simulink model "w3_warplab_trigger_proc"  (Simulink 7.7)
settings: Solver=ode45  StartTime=0.0  StopTime=100  RelTol=1e-3
InitFcn:
  | warplab_trigger_proc_init
StartFcn:
  | warplab_trigger_proc_init
undefined symbols (not defined in the file or in its folder): gcbh, xlBlockLoadCallback, xlGetNormalizedPeriod
libraries: xbsIndex_r4 x817, xbsEDKLib_r4 x1
(part 5 of 6)

== system w3_warplab_trigger_proc/Trigger Sources/Energy ==
  16LSB : xbsIndex_r4/Slice  nbits=16  boolean_output=off  mode=Lower Bit Location + Width  bit1=0  base1=MSB of Input  bit0=0  base0=LSB of Input  dbl_ovrd=off  block_type=slice
  16MSB : xbsIndex_r4/Slice  nbits=16  boolean_output=off  mode=Lower Bit Location + Width  bit1=0  base1=MSB of Input  bit0=16  base0=LSB of Input  dbl_ovrd=off  block_type=slice
  AntA Detector : Subsystem
  AntB Detector : Subsystem
  AntC Detector : Subsystem
  AntD Detector : Subsystem
  Convert : xbsIndex_r4/Convert  gui_display_data_type=Boolean  arith_type=Boolean  n_bits=16  bin_pt=14  float_type=Single  exp_bits=8  fraction_bits=24  quantization=Truncate  overflow=Wrap  en=off  latency=0  dbl_ovrd=off  pipeline=off  block_type=convert
  MIMO Logic : Subsystem
  Posedge : Subsystem
  RFA_RSSI : xbsIndex_r4/Gateway In  gui_display_data_type=Fixed-point  arith_type=Unsigned  n_bits=10  bin_pt=0  preci_type=Single  exp_width=8  frac_width=24  quantization=Truncate  overflow=Wrap  period=1  dbl_ovrd=off  timing_constraint=None  locs_specified=off  LOCs={}  UseAsADC=off  ADCChannel='1'  inherit_from_input=off  hdl_port=on  block_type=gatewayin
      settings: block_version=VER_STRING_GOES_HERE
  RFB_RSSI : xbsIndex_r4/Gateway In  gui_display_data_type=Fixed-point  arith_type=Unsigned  n_bits=10  bin_pt=0  preci_type=Single  exp_width=8  frac_width=24  quantization=Truncate  overflow=Wrap  period=1  dbl_ovrd=off  timing_constraint=None  locs_specified=off  LOCs={}  UseAsADC=off  ADCChannel='1'  inherit_from_input=off  hdl_port=on  block_type=gatewayin
      settings: infoedit="Gateway in block.  Converts inputs of type Simulink integer, double and fixed point to  Xilinx fixed point type.<P><P>Hardware notes:  In hardware these blocks become top level input ports."  block_version=VER_STRING_GOES_HERE
  RFC_RSSI : xbsIndex_r4/Gateway In  gui_display_data_type=Fixed-point  arith_type=Unsigned  n_bits=10  bin_pt=0  preci_type=Single  exp_width=8  frac_width=24  quantization=Truncate  overflow=Wrap  period=1  dbl_ovrd=off  timing_constraint=None  locs_specified=off  LOCs={}  UseAsADC=off  ADCChannel='1'  inherit_from_input=off  hdl_port=on  block_type=gatewayin
      settings: infoedit="Gateway in block.  Converts inputs of type Simulink integer, double and fixed point to  Xilinx fixed point type.<P><P>Hardware notes:  In hardware these blocks become top level input ports."  block_version=VER_STRING_GOES_HERE
  RFD_RSSI : xbsIndex_r4/Gateway In  gui_display_data_type=Fixed-point  arith_type=Unsigned  n_bits=10  bin_pt=0  preci_type=Single  exp_width=8  frac_width=24  quantization=Truncate  overflow=Wrap  period=1  dbl_ovrd=off  timing_constraint=None  locs_specified=off  LOCs={}  UseAsADC=off  ADCChannel='1'  inherit_from_input=off  hdl_port=on  block_type=gatewayin
      settings: infoedit="Gateway in block.  Converts inputs of type Simulink integer, double and fixed point to  Xilinx fixed point type.<P><P>Hardware notes:  In hardware these blocks become top level input ports."  block_version=VER_STRING_GOES_HERE
  RSSI_CLK : xbsIndex_r4/Gateway In  gui_display_data_type=Boolean  arith_type=Boolean  n_bits=10  bin_pt=0  preci_type=Single  exp_width=8  frac_width=24  quantization=Truncate  overflow=Wrap  period=1  dbl_ovrd=off  timing_constraint=None  locs_specified=off  LOCs={}  UseAsADC=off  ADCChannel='1'  inherit_from_input=off  hdl_port=on  block_type=gatewayin
      settings: block_version=VER_STRING_GOES_HERE
  b0 : xbsIndex_r4/Slice  nbits=1  boolean_output=off  mode=Lower Bit Location + Width  bit1=0  base1=MSB of Input  bit0=0  base0=LSB of Input  dbl_ovrd=off  block_type=slice
  b1 : xbsIndex_r4/Slice  nbits=1  boolean_output=off  mode=Lower Bit Location + Width  bit1=0  base1=MSB of Input  bit0=1  base0=LSB of Input  dbl_ovrd=off  block_type=slice
  b2 : xbsIndex_r4/Slice  nbits=1  boolean_output=off  mode=Lower Bit Location + Width  bit1=0  base1=MSB of Input  bit0=2  base0=LSB of Input  dbl_ovrd=off  block_type=slice
  b3 : xbsIndex_r4/Slice  nbits=1  boolean_output=off  mode=Lower Bit Location + Width  bit1=0  base1=MSB of Input  bit0=3  base0=LSB of Input  dbl_ovrd=off  block_type=slice
  b4 : xbsIndex_r4/Slice  nbits=1  boolean_output=off  mode=Lower Bit Location + Width  bit1=0  base1=MSB of Input  bit0=4  base0=LSB of Input  dbl_ovrd=off  block_type=slice
  b5 : xbsIndex_r4/Slice  nbits=1  boolean_output=off  mode=Lower Bit Location + Width  bit1=0  base1=MSB of Input  bit0=5  base0=LSB of Input  dbl_ovrd=off  block_type=slice
  b[15:8] : xbsIndex_r4/Slice  nbits=8  boolean_output=off  mode=Lower Bit Location + Width  bit1=0  base1=MSB of Input  bit0=8  base0=LSB of Input  dbl_ovrd=off  block_type=slice
  b[20:16] : xbsIndex_r4/Slice  nbits=5  boolean_output=off  mode=Lower Bit Location + Width  bit1=0  base1=MSB of Input  bit0=16  base0=LSB of Input  dbl_ovrd=off  block_type=slice
  b[7:0] : xbsIndex_r4/Slice  nbits=8  boolean_output=off  mode=Lower Bit Location + Width  bit1=0  base1=MSB of Input  bit0=0  base0=LSB of Input  dbl_ovrd=off  block_type=slice
  Trigger : Outport
  tag scope: pktDetMask_A=global, pktDetMask_B=global, pktDetMask_C=global, pktDetMask_D=global, pktDetReset=global, pktDet_duration_busy=global, pktDet_duration_idle=global, pktDet_energyThresh_busy=global, pktDet_energyThresh_idle=global, regPktDet_RSSIavgLength=global
  wires:
  AntA Detector/1(pktdet) -> MIMO Logic/1(Det A)
  [pktDetReset] -> Convert/1
  RFA_RSSI/1 -> AntA Detector/1(RSSI)
  [reg_pkt_det_config] -> b0/1, b1/1, b2/1, b3/1, b4/1, b5/1
  b0/1 -> [pktDetReset]
  b2/1 -> [pktDetMask_A]
  b3/1 -> [pktDetMask_B]
  [reg_pkt_det_thresh] -> 16LSB/1, 16MSB/1
  [reg_pkt_det_duration] -> b[7:0]/1, b[15:8]/1, b[20:16]/1
  16LSB/1 -> [pktDet_energyThresh_idle]
  16MSB/1 -> [pktDet_energyThresh_busy]
  b[7:0]/1 -> [pktDet_duration_idle]
  b[15:8]/1 -> [pktDet_duration_busy]
  b[20:16]/1 -> [regPktDet_RSSIavgLength]
  AntB Detector/1(pktdet) -> MIMO Logic/2(Det B)
  AntC Detector/1(pktdet) -> MIMO Logic/3(Det C)
  AntD Detector/1(pktdet) -> MIMO Logic/4(Det D)
  RFB_RSSI/1 -> AntB Detector/1(RSSI)
  RFC_RSSI/1 -> AntC Detector/1(RSSI)
  RFD_RSSI/1 -> AntD Detector/1(RSSI)
  Convert/1 -> AntA Detector/2(Reset), AntB Detector/2(Reset), AntC Detector/2(Reset), AntD Detector/2(Reset)
  b4/1 -> [pktDetMask_C]
  b5/1 -> [pktDetMask_D]
  MIMO Logic/1(PktDet) -> Trigger/1
  RSSI_CLK/1 -> Posedge/1(D)
  Posedge/1(Q) -> AntC Detector/3(En), AntD Detector/3(En), AntB Detector/3(En), AntA Detector/3(En)

== system w3_warplab_trigger_proc/Trigger Sources/Ethernet ==
  AXI_STR_TDATA : xbsIndex_r4/Gateway In  gui_display_data_type=Fixed-point  arith_type=Unsigned  n_bits=32  bin_pt=0  preci_type=Single  exp_width=8  frac_width=24  quantization="Round  (unbiased: +/- Inf)"  overflow=Wrap  period=1  dbl_ovrd=off  timing_constraint=None  locs_specified=off  LOCs={}  UseAsADC=off  ADCChannel='1'  inherit_from_input=off  hdl_port=on  block_type=gatewayin
  AXI_STR_TDEST : xbsIndex_r4/Gateway In  gui_display_data_type=Fixed-point  arith_type=Unsigned  n_bits=4  bin_pt=0  preci_type=Single  exp_width=8  frac_width=24  quantization="Round  (unbiased: +/- Inf)"  overflow=Wrap  period=1  dbl_ovrd=off  timing_constraint=None  locs_specified=off  LOCs={}  UseAsADC=off  ADCChannel='1'  inherit_from_input=off  hdl_port=on  block_type=gatewayin
  AXI_STR_TKEEP : xbsIndex_r4/Gateway In  gui_display_data_type=Fixed-point  arith_type=Unsigned  n_bits=4  bin_pt=0  preci_type=Single  exp_width=8  frac_width=24  quantization="Round  (unbiased: +/- Inf)"  overflow=Wrap  period=1  dbl_ovrd=off  timing_constraint=None  locs_specified=off  LOCs={}  UseAsADC=off  ADCChannel='1'  inherit_from_input=off  hdl_port=on  block_type=gatewayin
  AXI_STR_TLAST : xbsIndex_r4/Gateway In  gui_display_data_type=Fixed-point  arith_type=Unsigned  n_bits=1  bin_pt=0  preci_type=Single  exp_width=8  frac_width=24  quantization="Round  (unbiased: +/- Inf)"  overflow=Wrap  period=1  dbl_ovrd=off  timing_constraint=None  locs_specified=off  LOCs={}  UseAsADC=off  ADCChannel='1'  inherit_from_input=off  hdl_port=on  block_type=gatewayin
  AXI_STR_TREADY : xbsIndex_r4/Gateway In  gui_display_data_type=Fixed-point  arith_type=Unsigned  n_bits=1  bin_pt=0  preci_type=Single  exp_width=8  frac_width=24  quantization="Round  (unbiased: +/- Inf)"  overflow=Wrap  period=1  dbl_ovrd=off  timing_constraint=None  locs_specified=off  LOCs={}  UseAsADC=off  ADCChannel='1'  inherit_from_input=off  hdl_port=on  block_type=gatewayin
  AXI_STR_TSTRB : xbsIndex_r4/Gateway In  gui_display_data_type=Fixed-point  arith_type=Unsigned  n_bits=4  bin_pt=0  preci_type=Single  exp_width=8  frac_width=24  quantization="Round  (unbiased: +/- Inf)"  overflow=Wrap  period=1  dbl_ovrd=off  timing_constraint=None  locs_specified=off  LOCs={}  UseAsADC=off  ADCChannel='1'  inherit_from_input=off  hdl_port=on  block_type=gatewayin
  AXI_STR_TVALID : xbsIndex_r4/Gateway In  gui_display_data_type=Fixed-point  arith_type=Unsigned  n_bits=1  bin_pt=0  preci_type=Single  exp_width=8  frac_width=24  quantization="Round  (unbiased: +/- Inf)"  overflow=Wrap  period=1  dbl_ovrd=off  timing_constraint=None  locs_specified=off  LOCs={}  UseAsADC=off  ADCChannel='1'  inherit_from_input=off  hdl_port=on  block_type=gatewayin
  Constant{,1..4,6..7} (7 alike) : Constant  Value=0
  Pkt Comp : Subsystem
  Terminator : Terminator
  Terminator1 : Terminator
  Terminator2 : Terminator
  Trigger : Outport
  wires:
  Constant/1 -> AXI_STR_TVALID/1
  Constant1/1 -> AXI_STR_TDATA/1
  Constant2/1 -> AXI_STR_TLAST/1
  Constant3/1 -> AXI_STR_TSTRB/1
  AXI_STR_TVALID/1 -> Pkt Comp/1(TVALID)  "TVALID"
  AXI_STR_TDATA/1 -> Pkt Comp/2(TDATA)  "TDATA"
  AXI_STR_TREADY/1 -> Pkt Comp/3(TREADY)  "TREADY"
  Constant4/1 -> AXI_STR_TREADY/1
  AXI_STR_TLAST/1 -> Pkt Comp/4(TLAST)  "TLAST"
  Constant6/1 -> AXI_STR_TKEEP/1
  Constant7/1 -> AXI_STR_TDEST/1
  AXI_STR_TDEST/1 -> Terminator2/1  "TDEST"
  AXI_STR_TKEEP/1 -> Terminator1/1  "TKEEP"
  AXI_STR_TSTRB/1 -> Terminator/1  "TSTRB"
  Pkt Comp/1(Trigger) -> Trigger/1

== system w3_warplab_trigger_proc/Trigger Sources/Software ==
  Trigger : Outport
  wires:
  [Software_Trig] -> Trigger/1

== system w3_warplab_trigger_proc/Trigger Sources/Energy/AntA Detector ==
  RSSI : Inport
  Reset : Inport  Port=2
  En : Inport  Port=3
  ASR : xbsIndex_r4/Addressable Shift Register  infer_latency=on  depth=2  initVector=[0]  en=on  dbl_ovrd=off  use_behavioral_HDL=off  Optimization=Resource  use_rpm=off  block_type=addrsr
      settings: infoedit="Delay of configurable length.  Any element in the delay line can be addressed and driven onto the output port.<br><br>Hardware notes: This block is implemented using SRL16s. If Virtex-4 or Spartan-3 device is used, multiple SRLC16s are cascaded together."  block_version=VER_STRING_GOES_HERE
  Busy Detection : Subsystem
  Delay : xbsIndex_r4/Delay  rst=off  infoeditControl=Selection of Reset will increase slice count due to use of real FFs and instead of SRLs  en=off  latency=2  dbl_ovrd=off  reg_retiming=off  block_type=delay
  Gateway Out{,1..5} (6 alike) : xbsIndex_r4/Gateway Out  inherit_from_input=off  hdl_port=off  timing_constraint=None  locs_specified=off  LOCs={}  UseAsDAC=off  DACChannel='1'  block_type=gatewayout
      settings: infoedit="Gateway out block.  Converts Xilinx fixed point inputs into ouputs of type Simulink integer, double, or fixed point.<P><P>Hardware notes:  In hardware these blocks become top level output ports or are discarded, depending on how they are configured."  block_version=8.2
  Idle Detection : Subsystem
  Logical : xbsIndex_r4/Logical  logical_function=AND  inputs=2  en=off  latency=0  precision=Full  arith_type=Unsigned  n_bits=16  bin_pt=0  align_bp=on  dbl_ovrd=off  block_type=logical
  Pkt Det Decision : Scope  NumInputPorts=6
      settings: TimeRange=1000  YMin=0~0~0~0~0~0  YMax=1000~15000~1~1~1~1
  Running Sum : Subsystem
  pktdet : Outport
  wires:
  Reset/1 -> Running Sum/2(reset), Idle Detection/2(Reset), Busy Detection/2(Reset)
  [regPktDet_RSSIavgLength] -> Running Sum/3(avglen)
  Gateway Out/1 -> Pkt Det Decision/1  "RAWRSSI"
  Gateway Out1/1 -> Pkt Det Decision/2  "AVGRSSI"
  Gateway Out2/1 -> Pkt Det Decision/3  "IDLE"
  RSSI/1 -> Running Sum/1(RSSI), Gateway Out/1
  Running Sum/1(avg) -> Idle Detection/1(Avg RSSI), Busy Detection/1(Avg RSSI), Gateway Out1/1
  Idle Detection/1(Idle) -> Gateway Out2/1, Delay/1
  [pktDet_duration_busy] -> ASR/2
  ASR/1 -> Logical/1, Gateway Out5/1
  Busy Detection/1(Busy) -> Logical/2, Gateway Out3/1
  Logical/1 -> pktdet/1, Gateway Out4/1
  Gateway Out3/1 -> Pkt Det Decision/5  "BUSY"
  Gateway Out4/1 -> Pkt Det Decision/6  "DET"
  Gateway Out5/1 -> Pkt Det Decision/4  "IDLE DLY"
  Delay/1 -> ASR/1
  En/1 -> Running Sum/4(en), ASR/3, Idle Detection/3(en), Busy Detection/3(en)

== system w3_warplab_trigger_proc/Trigger Sources/Energy/AntB Detector ==
  RSSI : Inport
  Reset : Inport  Port=2
  En : Inport  Port=3
  ASR : xbsIndex_r4/Addressable Shift Register  infer_latency=on  depth=2  initVector=[0]  en=on  dbl_ovrd=off  use_behavioral_HDL=off  Optimization=Resource  use_rpm=off  block_type=addrsr
      settings: infoedit="Delay of configurable length.  Any element in the delay line can be addressed and driven onto the output port.<br><br>Hardware notes: This block is implemented using SRL16s. If Virtex-4 or Spartan-3 device is used, multiple SRLC16s are cascaded together."  block_version=VER_STRING_GOES_HERE
  Busy Detection : Subsystem
  Delay : xbsIndex_r4/Delay  rst=off  infoeditControl=Selection of Reset will increase slice count due to use of real FFs and instead of SRLs  en=off  latency=2  dbl_ovrd=off  reg_retiming=off  block_type=delay
  Gateway Out{,1..5} (6 alike) : xbsIndex_r4/Gateway Out  inherit_from_input=off  hdl_port=off  timing_constraint=None  locs_specified=off  LOCs={}  UseAsDAC=off  DACChannel='1'  block_type=gatewayout
      settings: infoedit="Gateway out block.  Converts Xilinx fixed point inputs into ouputs of type Simulink integer, double, or fixed point.<P><P>Hardware notes:  In hardware these blocks become top level output ports or are discarded, depending on how they are configured."  block_version=8.2
  Idle Detection : Subsystem
  Logical : xbsIndex_r4/Logical  logical_function=AND  inputs=2  en=off  latency=0  precision=Full  arith_type=Unsigned  n_bits=16  bin_pt=0  align_bp=on  dbl_ovrd=off  block_type=logical
  Pkt Det Decision : Scope  NumInputPorts=6
      settings: TimeRange=1000  YMin=0~0~0~0~0~0  YMax=1000~15000~1~1~1~1
  Running Sum : Subsystem
  pktdet : Outport
  wires:
  En/1 -> ASR/3, Idle Detection/3(en), Busy Detection/3(en), Running Sum/4(en)
  Delay/1 -> ASR/1
  Gateway Out5/1 -> Pkt Det Decision/4  "IDLE DLY"
  Gateway Out4/1 -> Pkt Det Decision/6  "DET"
  Gateway Out3/1 -> Pkt Det Decision/5  "BUSY"
  Logical/1 -> Gateway Out4/1, pktdet/1
  Busy Detection/1(Busy) -> Gateway Out3/1, Logical/2
  ASR/1 -> Gateway Out5/1, Logical/1
  [pktDet_duration_busy] -> ASR/2
  Idle Detection/1(Idle) -> Delay/1, Gateway Out2/1
  Running Sum/1(avg) -> Gateway Out1/1, Idle Detection/1(Avg RSSI), Busy Detection/1(Avg RSSI)
  RSSI/1 -> Gateway Out/1, Running Sum/1(RSSI)
  Gateway Out2/1 -> Pkt Det Decision/3  "IDLE"
  Gateway Out1/1 -> Pkt Det Decision/2  "AVGRSSI"
  Gateway Out/1 -> Pkt Det Decision/1  "RAWRSSI"
  [regPktDet_RSSIavgLength] -> Running Sum/3(avglen)
  Reset/1 -> Idle Detection/2(Reset), Busy Detection/2(Reset), Running Sum/2(reset)

== system w3_warplab_trigger_proc/Trigger Sources/Energy/AntC Detector ==
  RSSI : Inport
  Reset : Inport  Port=2
  En : Inport  Port=3
  ASR : xbsIndex_r4/Addressable Shift Register  infer_latency=on  depth=2  initVector=[0]  en=on  dbl_ovrd=off  use_behavioral_HDL=off  Optimization=Resource  use_rpm=off  block_type=addrsr
      settings: infoedit="Delay of configurable length.  Any element in the delay line can be addressed and driven onto the output port.<br><br>Hardware notes: This block is implemented using SRL16s. If Virtex-4 or Spartan-3 device is used, multiple SRLC16s are cascaded together."  block_version=VER_STRING_GOES_HERE
  Busy Detection : Subsystem
  Delay : xbsIndex_r4/Delay  rst=off  infoeditControl=Selection of Reset will increase slice count due to use of real FFs and instead of SRLs  en=off  latency=2  dbl_ovrd=off  reg_retiming=off  block_type=delay
  Gateway Out{,1..5} (6 alike) : xbsIndex_r4/Gateway Out  inherit_from_input=off  hdl_port=off  timing_constraint=None  locs_specified=off  LOCs={}  UseAsDAC=off  DACChannel='1'  block_type=gatewayout
      settings: infoedit="Gateway out block.  Converts Xilinx fixed point inputs into ouputs of type Simulink integer, double, or fixed point.<P><P>Hardware notes:  In hardware these blocks become top level output ports or are discarded, depending on how they are configured."  block_version=8.2
  Idle Detection : Subsystem
  Logical : xbsIndex_r4/Logical  logical_function=AND  inputs=2  en=off  latency=0  precision=Full  arith_type=Unsigned  n_bits=16  bin_pt=0  align_bp=on  dbl_ovrd=off  block_type=logical
  Pkt Det Decision : Scope  NumInputPorts=6
      settings: TimeRange=1000  YMin=0~0~0~0~0~0  YMax=1000~15000~1~1~1~1
  Running Sum : Subsystem
  pktdet : Outport
  wires:
  Reset/1 -> Running Sum/2(reset), Busy Detection/2(Reset), Idle Detection/2(Reset)
  [regPktDet_RSSIavgLength] -> Running Sum/3(avglen)
  Gateway Out/1 -> Pkt Det Decision/1  "RAWRSSI"
  Gateway Out1/1 -> Pkt Det Decision/2  "AVGRSSI"
  Gateway Out2/1 -> Pkt Det Decision/3  "IDLE"
  RSSI/1 -> Running Sum/1(RSSI), Gateway Out/1
  Running Sum/1(avg) -> Busy Detection/1(Avg RSSI), Idle Detection/1(Avg RSSI), Gateway Out1/1
  Idle Detection/1(Idle) -> Gateway Out2/1, Delay/1
  [pktDet_duration_busy] -> ASR/2
  ASR/1 -> Logical/1, Gateway Out5/1
  Busy Detection/1(Busy) -> Logical/2, Gateway Out3/1
  Logical/1 -> pktdet/1, Gateway Out4/1
  Gateway Out3/1 -> Pkt Det Decision/5  "BUSY"
  Gateway Out4/1 -> Pkt Det Decision/6  "DET"
  Gateway Out5/1 -> Pkt Det Decision/4  "IDLE DLY"
  Delay/1 -> ASR/1
  En/1 -> Running Sum/4(en), ASR/3, Busy Detection/3(en), Idle Detection/3(en)

== system w3_warplab_trigger_proc/Trigger Sources/Energy/AntD Detector ==
  RSSI : Inport
  Reset : Inport  Port=2
  En : Inport  Port=3
  ASR : xbsIndex_r4/Addressable Shift Register  infer_latency=on  depth=2  initVector=[0]  en=on  dbl_ovrd=off  use_behavioral_HDL=off  Optimization=Resource  use_rpm=off  block_type=addrsr
      settings: infoedit="Delay of configurable length.  Any element in the delay line can be addressed and driven onto the output port.<br><br>Hardware notes: This block is implemented using SRL16s. If Virtex-4 or Spartan-3 device is used, multiple SRLC16s are cascaded together."  block_version=VER_STRING_GOES_HERE
  Busy Detection : Subsystem
  Delay : xbsIndex_r4/Delay  rst=off  infoeditControl=Selection of Reset will increase slice count due to use of real FFs and instead of SRLs  en=off  latency=2  dbl_ovrd=off  reg_retiming=off  block_type=delay
  Gateway Out{,1..5} (6 alike) : xbsIndex_r4/Gateway Out  inherit_from_input=off  hdl_port=off  timing_constraint=None  locs_specified=off  LOCs={}  UseAsDAC=off  DACChannel='1'  block_type=gatewayout
      settings: infoedit="Gateway out block.  Converts Xilinx fixed point inputs into ouputs of type Simulink integer, double, or fixed point.<P><P>Hardware notes:  In hardware these blocks become top level output ports or are discarded, depending on how they are configured."  block_version=8.2
  Idle Detection : Subsystem
  Logical : xbsIndex_r4/Logical  logical_function=AND  inputs=2  en=off  latency=0  precision=Full  arith_type=Unsigned  n_bits=16  bin_pt=0  align_bp=on  dbl_ovrd=off  block_type=logical
  Pkt Det Decision : Scope  NumInputPorts=6
      settings: TimeRange=1000  YMin=0~0~0~0~0~0  YMax=1000~15000~1~1~1~1
  Running Sum : Subsystem
  pktdet : Outport
  wires:
  En/1 -> ASR/3, Idle Detection/3(en), Busy Detection/3(en), Running Sum/4(en)
  Delay/1 -> ASR/1
  Gateway Out5/1 -> Pkt Det Decision/4  "IDLE DLY"
  Gateway Out4/1 -> Pkt Det Decision/6  "DET"
  Gateway Out3/1 -> Pkt Det Decision/5  "BUSY"
  Logical/1 -> Gateway Out4/1, pktdet/1
  Busy Detection/1(Busy) -> Gateway Out3/1, Logical/2
  ASR/1 -> Gateway Out5/1, Logical/1
  [pktDet_duration_busy] -> ASR/2
  Idle Detection/1(Idle) -> Delay/1, Gateway Out2/1
  Running Sum/1(avg) -> Gateway Out1/1, Idle Detection/1(Avg RSSI), Busy Detection/1(Avg RSSI)
  RSSI/1 -> Gateway Out/1, Running Sum/1(RSSI)
  Gateway Out2/1 -> Pkt Det Decision/3  "IDLE"
  Gateway Out1/1 -> Pkt Det Decision/2  "AVGRSSI"
  Gateway Out/1 -> Pkt Det Decision/1  "RAWRSSI"
  [regPktDet_RSSIavgLength] -> Running Sum/3(avglen)
  Reset/1 -> Idle Detection/2(Reset), Busy Detection/2(Reset), Running Sum/2(reset)

== system w3_warplab_trigger_proc/Trigger Sources/Energy/MIMO Logic ==
  Det A : Inport
  Det B : Inport  Port=2
  Det C : Inport  Port=3
  Det D : Inport  Port=4
  Convert{1..8} (8 alike) : xbsIndex_r4/Convert  gui_display_data_type=Fixed-point  arith_type=Unsigned  n_bits=1  bin_pt=0  float_type=Single  exp_bits=8  fraction_bits=24  quantization=Truncate  overflow=Flag as error  en=off  latency=0  dbl_ovrd=off  pipeline=off  block_type=convert
      settings: block_version=10.1.3
  Logical{,1,3..4} (4 alike) : xbsIndex_r4/Logical  logical_function=AND  inputs=2  en=off  latency=0  precision=Full  arith_type=Unsigned  n_bits=16  bin_pt=0  align_bp=on  dbl_ovrd=off  block_type=logical
  Logical2 : xbsIndex_r4/Logical  logical_function=OR  inputs=4  en=off  latency=0  precision=Full  arith_type=Unsigned  n_bits=16  bin_pt=0  align_bp=on  dbl_ovrd=off  block_type=logical
  PktDet : Outport
  wires:
  [pktDetMask_A] -> Convert2/1
  [pktDetMask_B] -> Convert3/1
  Det A/1 -> Convert7/1
  Det B/1 -> Convert1/1
  Convert7/1 -> Logical/1
  Convert2/1 -> Logical/2
  Convert1/1 -> Logical1/1
  Convert3/1 -> Logical1/2
  Logical/1 -> Logical2/1
  Logical1/1 -> Logical2/2
  Logical2/1 -> PktDet/1
  [pktDetMask_C] -> Convert5/1
  Det C/1 -> Convert4/1
  Convert4/1 -> Logical3/1
  Convert5/1 -> Logical3/2
  Logical3/1 -> Logical2/3
  [pktDetMask_D] -> Convert8/1
  Det D/1 -> Convert6/1
  Convert6/1 -> Logical4/1
  Convert8/1 -> Logical4/2
  Logical4/1 -> Logical2/4

== system w3_warplab_trigger_proc/Trigger Sources/Energy/Posedge ==
  D : Inport
  Delay : xbsIndex_r4/Delay  rst=off  infoeditControl=Selection of Reset will increase slice count due to use of real FFs and instead of SRLs  en=off  latency=1  dbl_ovrd=off  reg_retiming=off  block_type=delay
      settings: infoedit=Hardware notes: A delay line is a chain, each link of which is an SRL16 followed by a flip-flop. If register retiming is enabled, the delay line is a chain of flip-flops.  block_version=8.2
  Inverter : xbsIndex_r4/Inverter  en=off  latency=0  dbl_ovrd=off  block_type=inv
      settings: block_version=8.2
  Logical : xbsIndex_r4/Logical  logical_function=AND  inputs=2  en=off  latency=0  precision=Full  arith_type=Unsigned  n_bits=16  bin_pt=0  align_bp=on  dbl_ovrd=off  block_type=logical
      settings: block_version=8.2
  Q : Outport
  wires:
  D/1 -> Inverter/1, Logical/1
  Inverter/1 -> Delay/1
  Delay/1 -> Logical/2
  Logical/1 -> Q/1

== system w3_warplab_trigger_proc/Trigger Sources/Ethernet/Pkt Comp ==
  TVALID : Inport
  TDATA : Inport  Port=2
  TREADY : Inport  Port=3
  TLAST : Inport  Port=4
  Convert2 : xbsIndex_r4/Convert  gui_display_data_type=Boolean  arith_type=Boolean  n_bits=16  bin_pt=14  float_type=Single  exp_bits=8  fraction_bits=24  quantization=Truncate  overflow=Wrap  en=off  latency=0  dbl_ovrd=off  pipeline=off  block_type=convert
  Convert3 : xbsIndex_r4/Convert  gui_display_data_type=Boolean  arith_type=Boolean  n_bits=16  bin_pt=14  float_type=Single  exp_bits=8  fraction_bits=24  quantization=Truncate  overflow=Wrap  en=off  latency=0  dbl_ovrd=off  pipeline=off  block_type=convert
  Delay : xbsIndex_r4/Delay  rst=off  infoeditControl=Selection of Reset will increase slice count due to use of real FFs and instead of SRLs  en=off  latency=4  dbl_ovrd=off  reg_retiming=off  block_type=delay
  Delay1 : xbsIndex_r4/Delay  rst=off  infoeditControl=Selection of Reset will increase slice count due to use of real FFs and instead of SRLs  en=off  latency=3  dbl_ovrd=off  reg_retiming=off  block_type=delay
  Delay2 : xbsIndex_r4/Delay  rst=off  infoeditControl=Selection of Reset will increase slice count due to use of real FFs and instead of SRLs  en=off  latency=1  dbl_ovrd=off  reg_retiming=off  block_type=delay
  Delay3 : xbsIndex_r4/Delay  rst=off  infoeditControl=Selection of Reset will increase slice count due to use of real FFs and instead of SRLs  en=off  latency=1  dbl_ovrd=off  reg_retiming=off  block_type=delay
  Logical : xbsIndex_r4/Logical  logical_function=AND  inputs=2  en=off  latency=0  precision=Full  arith_type=Unsigned  n_bits=16  bin_pt=0  align_bp=on  dbl_ovrd=off  block_type=logical
  Output Reg 0 : Subsystem
  Pkt Match : Subsystem
  Pkt Word Addr : xbsIndex_r4/Counter  cnt_type=Count Limited  cnt_to=63  operation=Up  start_count=0  cnt_by_val=1  arith_type=Unsigned  n_bits=6  bin_pt=0  load_pin=off  rst=on  en=on  explicit_period=off  period=1  dbl_ovrd=off  use_behavioral_HDL=off  implementation=Fabric  block_type=counter
  Word Comp 0 : Subsystem
  Trigger : Outport
  tag scope: WordMatch_0=global
  wires:
  Logical/1 -> Convert2/1
  TVALID/1 -> Logical/1
  TREADY/1 -> Logical/2
  Pkt Word Addr/1 -> Word Comp 0/1(Word Addr)
  TLAST/1 -> Convert3/1
  Convert2/1 -> Pkt Word Addr/2, Delay3/1
  Convert3/1 -> Pkt Word Addr/1, Delay/1, Delay1/1
  TDATA/1 -> Delay2/1
  Delay/1 -> Pkt Match/3(Reset)
  Word Comp 0/1(Word Match) -> Pkt Match/2(Word Match), [WordMatch_0]
  Delay1/1 -> Output Reg 0/2(Done)
  Pkt Match/1(Pkt Match) -> Output Reg 0/1(Match)
  Output Reg 0/1(Out) -> Trigger/1
  Delay2/1 -> Word Comp 0/2(TDATA)
  Delay3/1 -> Pkt Match/1(Valid)

== system w3_warplab_trigger_proc/Trigger Sources/Energy/AntA Detector/Busy Detection ==
  Avg RSSI : Inport
  Reset : Inport  Port=2
  en : Inport  Port=3
  Convert1 : xbsIndex_r4/Convert  gui_display_data_type=Fixed-point  arith_type=Unsigned  n_bits=1  bin_pt=0  float_type=Single  exp_bits=8  fraction_bits=24  quantization=Truncate  overflow=Wrap  en=off  latency=0  dbl_ovrd=off  pipeline=off  block_type=convert
      settings: block_version=VER_STRING_GOES_HERE
  Counter1 : xbsIndex_r4/Counter  cnt_type=Free Running  cnt_to=Inf  operation=Up  start_count=0  cnt_by_val=1  arith_type=Unsigned  n_bits=11  bin_pt=0  load_pin=off  rst=on  en=on  explicit_period=off  period=4  dbl_ovrd=off  use_behavioral_HDL=off  implementation=Fabric  use_rpm=off  block_type=counter
  Inverter1 : xbsIndex_r4/Inverter  en=off  latency=0  dbl_ovrd=off  block_type=inv
      settings: xl_area=[0 0 0 0 0 0 0]  block_version=8.2
  Logical : xbsIndex_r4/Logical  logical_function=AND  inputs=2  en=off  latency=0  precision=Full  arith_type=Unsigned  n_bits=16  bin_pt=0  align_bp=on  dbl_ovrd=off  block_type=logical
  Logical1 : xbsIndex_r4/Logical  logical_function=OR  inputs=2  en=off  latency=0  precision=Full  arith_type=Unsigned  n_bits=16  bin_pt=0  align_bp=on  dbl_ovrd=off  block_type=logical
  Relational2 : xbsIndex_r4/Relational  mode=a>b  en=off  latency=0  dbl_ovrd=off  block_type=relational
      settings: block_version=VER_STRING_GOES_HERE
  Relational3 : xbsIndex_r4/Relational  mode=a>b  en=off  latency=0  dbl_ovrd=off  block_type=relational
      settings: block_version=VER_STRING_GOES_HERE
  S-R Latch : Subsystem
  Busy : Outport
  wires:
  [pktDet_energyThresh_busy] -> Relational2/2
  Reset/1 -> Logical1/1
  Logical1/1 -> Counter1/1, S-R Latch/1(R)
  Inverter1/1 -> Logical1/2
  Counter1/1 -> Relational3/1
  [pktDet_duration_busy] -> Relational3/2
  Relational3/1 -> S-R Latch/2(S)
  S-R Latch/1(Q) -> Convert1/1
  Avg RSSI/1 -> Relational2/1
  Convert1/1 -> Busy/1
  Logical/1 -> Counter1/2
  Relational2/1 -> Logical/1, Inverter1/1
  en/1 -> Logical/2

== system w3_warplab_trigger_proc/Trigger Sources/Energy/AntA Detector/Idle Detection ==
  Avg RSSI : Inport
  Reset : Inport  Port=2
  en : Inport  Port=3
  Convert1 : xbsIndex_r4/Convert  gui_display_data_type=Fixed-point  arith_type=Unsigned  n_bits=1  bin_pt=0  float_type=Single  exp_bits=8  fraction_bits=24  quantization=Truncate  overflow=Wrap  en=off  latency=0  dbl_ovrd=off  pipeline=off  block_type=convert
      settings: block_version=VER_STRING_GOES_HERE
  Counter1 : xbsIndex_r4/Counter  cnt_type=Free Running  cnt_to=Inf  operation=Up  start_count=0  cnt_by_val=1  arith_type=Unsigned  n_bits=11  bin_pt=0  load_pin=off  rst=on  en=on  explicit_period=off  period=4  dbl_ovrd=off  use_behavioral_HDL=off  implementation=Fabric  use_rpm=off  block_type=counter
  Inverter1 : xbsIndex_r4/Inverter  en=off  latency=0  dbl_ovrd=off  block_type=inv
      settings: xl_area=[0 0 0 0 0 0 0]  block_version=8.2
  Logical : xbsIndex_r4/Logical  logical_function=AND  inputs=2  en=off  latency=0  precision=Full  arith_type=Unsigned  n_bits=16  bin_pt=0  align_bp=on  dbl_ovrd=off  block_type=logical
  Logical1 : xbsIndex_r4/Logical  logical_function=OR  inputs=2  en=off  latency=0  precision=Full  arith_type=Unsigned  n_bits=16  bin_pt=0  align_bp=on  dbl_ovrd=off  block_type=logical
  Relational2 : xbsIndex_r4/Relational  mode=a<b  en=off  latency=0  dbl_ovrd=off  block_type=relational
      settings: block_version=VER_STRING_GOES_HERE
  Relational3 : xbsIndex_r4/Relational  mode=a>b  en=off  latency=0  dbl_ovrd=off  block_type=relational
      settings: block_version=VER_STRING_GOES_HERE
  S-R Latch : Subsystem
  Idle : Outport
  wires:
  Convert1/1 -> Idle/1
  Avg RSSI/1 -> Relational2/1
  S-R Latch/1(Q) -> Convert1/1
  Relational3/1 -> S-R Latch/2(S)
  [pktDet_duration_idle] -> Relational3/2
  Counter1/1 -> Relational3/1
  Inverter1/1 -> Logical1/2
  Logical1/1 -> Counter1/1, S-R Latch/1(R)
  Reset/1 -> Logical1/1
  Relational2/1 -> Logical/1, Inverter1/1
  [pktDet_energyThresh_idle] -> Relational2/2
  en/1 -> Logical/2
  Logical/1 -> Counter1/2

== system w3_warplab_trigger_proc/Trigger Sources/Energy/AntA Detector/Running Sum ==
  note: This block impelemnts a variable-length running sum.
      | For a sum y(n) of the previous N samples of sequence x(n), it implements
      | y(n) = y(n-1) + x(n) - x(n-N)
      | This requires a careful reset procedure, where the full shift register
      | is zerored out. Otherwise the feedback-based sum stops working.
  RSSI : Inport
  reset : Inport  Port=2
  avglen : Inport  Port=3
  en : Inport  Port=4
  ASR : xbsIndex_r4/Addressable Shift Register  infer_latency=on  depth=2  initVector=[0]  en=on  dbl_ovrd=off  use_behavioral_HDL=off  Optimization=Resource  use_rpm=off  block_type=addrsr
      settings: infoedit="Delay of configurable length.  Any element in the delay line can be addressed and driven onto the output port.<br><br>Hardware notes: This block is implemented using SRL16s. If Virtex-4 or Spartan-3 device is used, multiple SRLC16s are cascaded together."  block_version=VER_STRING_GOES_HERE
  Accumulator : xbsIndex_r4/Accumulator  operation=Add  n_bits=17  overflow=Flag as error  scale=1  rst=on  infoeditControl=reset for floating point data type must be asserted for a minimum of 2 cycles  hasbypass=off  en=on  latency=0  dbl_ovrd=off  msb_inp=100  msb=100  lsb=-100  use_behavioral_HDL=on  implementation=Fabric  block_type=accum
      settings: block_version=VER_STRING_GOES_HERE
  AddSub : xbsIndex_r4/AddSub  mode=Subtraction  use_carryin=off  use_carryout=off  en=off  latency=0  precision=Full  arith_type=Unsigned  n_bits=10  bin_pt=0  quantization=Truncate  overflow=Wrap  dbl_ovrd=off  use_behavioral_HDL=off  hw_selection=Fabric  pipelined=off  use_rpm=on  block_type=addsub
      settings: block_version=VER_STRING_GOES_HERE
  Convert7 : xbsIndex_r4/Convert  gui_display_data_type=Fixed-point  arith_type=Unsigned  n_bits=17  bin_pt=0  float_type=Single  exp_bits=8  fraction_bits=24  quantization=Truncate  overflow=Saturate  en=off  latency=0  dbl_ovrd=off  pipeline=off  block_type=convert
      settings: block_version=10.1.3
  Logical : xbsIndex_r4/Logical  logical_function=OR  inputs=2  en=off  latency=0  precision=Full  arith_type=Unsigned  n_bits=16  bin_pt=0  align_bp=on  dbl_ovrd=off  block_type=logical
  Long Reset Gen : Subsystem
  Register : xbsIndex_r4/Register  init=0  rst=on  en=off  dbl_ovrd=off  block_type=register
      settings: block_version=VER_STRING_GOES_HERE
  avg : Outport
  wires:
  ASR/1 -> AddSub/2
  AddSub/1 -> Accumulator/1
  Register/1 -> ASR/1, AddSub/1
  avglen/1 -> ASR/2, Long Reset Gen/1(duration)
  RSSI/1 -> Register/1
  Accumulator/1 -> Convert7/1
  Logical/1 -> Register/2, Accumulator/2
  reset/1 -> Long Reset Gen/2(reset_in), Logical/2
  Long Reset Gen/1(reset_out) -> Logical/1
  Convert7/1 -> avg/1
  en/1 -> ASR/3, Accumulator/3

== system w3_warplab_trigger_proc/Trigger Sources/Energy/AntB Detector/Busy Detection ==
  Avg RSSI : Inport
  Reset : Inport  Port=2
  en : Inport  Port=3
  Convert1 : xbsIndex_r4/Convert  gui_display_data_type=Fixed-point  arith_type=Unsigned  n_bits=1  bin_pt=0  float_type=Single  exp_bits=8  fraction_bits=24  quantization=Truncate  overflow=Wrap  en=off  latency=0  dbl_ovrd=off  pipeline=off  block_type=convert
      settings: block_version=VER_STRING_GOES_HERE
  Counter1 : xbsIndex_r4/Counter  cnt_type=Free Running  cnt_to=Inf  operation=Up  start_count=0  cnt_by_val=1  arith_type=Unsigned  n_bits=11  bin_pt=0  load_pin=off  rst=on  en=on  explicit_period=off  period=4  dbl_ovrd=off  use_behavioral_HDL=off  implementation=Fabric  use_rpm=off  block_type=counter
  Inverter1 : xbsIndex_r4/Inverter  en=off  latency=0  dbl_ovrd=off  block_type=inv
      settings: xl_area=[0 0 0 0 0 0 0]  block_version=8.2
  Logical : xbsIndex_r4/Logical  logical_function=AND  inputs=2  en=off  latency=0  precision=Full  arith_type=Unsigned  n_bits=16  bin_pt=0  align_bp=on  dbl_ovrd=off  block_type=logical
  Logical1 : xbsIndex_r4/Logical  logical_function=OR  inputs=2  en=off  latency=0  precision=Full  arith_type=Unsigned  n_bits=16  bin_pt=0  align_bp=on  dbl_ovrd=off  block_type=logical
  Relational2 : xbsIndex_r4/Relational  mode=a>b  en=off  latency=0  dbl_ovrd=off  block_type=relational
      settings: block_version=VER_STRING_GOES_HERE
  Relational3 : xbsIndex_r4/Relational  mode=a>b  en=off  latency=0  dbl_ovrd=off  block_type=relational
      settings: block_version=VER_STRING_GOES_HERE
  S-R Latch : Subsystem
  Busy : Outport
  wires:
  [pktDet_energyThresh_busy] -> Relational2/2
  Reset/1 -> Logical1/1
  Logical1/1 -> Counter1/1, S-R Latch/1(R)
  Inverter1/1 -> Logical1/2
  Counter1/1 -> Relational3/1
  [pktDet_duration_busy] -> Relational3/2
  Relational3/1 -> S-R Latch/2(S)
  S-R Latch/1(Q) -> Convert1/1
  Avg RSSI/1 -> Relational2/1
  Convert1/1 -> Busy/1
  Logical/1 -> Counter1/2
  Relational2/1 -> Logical/1, Inverter1/1
  en/1 -> Logical/2

== system w3_warplab_trigger_proc/Trigger Sources/Energy/AntB Detector/Idle Detection ==
  Avg RSSI : Inport
  Reset : Inport  Port=2
  en : Inport  Port=3
  Convert1 : xbsIndex_r4/Convert  gui_display_data_type=Fixed-point  arith_type=Unsigned  n_bits=1  bin_pt=0  float_type=Single  exp_bits=8  fraction_bits=24  quantization=Truncate  overflow=Wrap  en=off  latency=0  dbl_ovrd=off  pipeline=off  block_type=convert
      settings: block_version=VER_STRING_GOES_HERE
  Counter1 : xbsIndex_r4/Counter  cnt_type=Free Running  cnt_to=Inf  operation=Up  start_count=0  cnt_by_val=1  arith_type=Unsigned  n_bits=11  bin_pt=0  load_pin=off  rst=on  en=on  explicit_period=off  period=4  dbl_ovrd=off  use_behavioral_HDL=off  implementation=Fabric  use_rpm=off  block_type=counter
  Inverter1 : xbsIndex_r4/Inverter  en=off  latency=0  dbl_ovrd=off  block_type=inv
      settings: xl_area=[0 0 0 0 0 0 0]  block_version=8.2
  Logical : xbsIndex_r4/Logical  logical_function=AND  inputs=2  en=off  latency=0  precision=Full  arith_type=Unsigned  n_bits=16  bin_pt=0  align_bp=on  dbl_ovrd=off  block_type=logical
  Logical1 : xbsIndex_r4/Logical  logical_function=OR  inputs=2  en=off  latency=0  precision=Full  arith_type=Unsigned  n_bits=16  bin_pt=0  align_bp=on  dbl_ovrd=off  block_type=logical
  Relational2 : xbsIndex_r4/Relational  mode=a<b  en=off  latency=0  dbl_ovrd=off  block_type=relational
      settings: block_version=VER_STRING_GOES_HERE
  Relational3 : xbsIndex_r4/Relational  mode=a>b  en=off  latency=0  dbl_ovrd=off  block_type=relational
      settings: block_version=VER_STRING_GOES_HERE
  S-R Latch : Subsystem
  Idle : Outport
  wires:
  Convert1/1 -> Idle/1
  Avg RSSI/1 -> Relational2/1
  S-R Latch/1(Q) -> Convert1/1
  Relational3/1 -> S-R Latch/2(S)
  [pktDet_duration_idle] -> Relational3/2
  Counter1/1 -> Relational3/1
  Inverter1/1 -> Logical1/2
  Logical1/1 -> Counter1/1, S-R Latch/1(R)
  Reset/1 -> Logical1/1
  Relational2/1 -> Logical/1, Inverter1/1
  [pktDet_energyThresh_idle] -> Relational2/2
  en/1 -> Logical/2
  Logical/1 -> Counter1/2

== system w3_warplab_trigger_proc/Trigger Sources/Energy/AntB Detector/Running Sum ==
  note: This block impelemnts a variable-length running sum.
      | For a sum y(n) of the previous N samples of sequence x(n), it implements
      | y(n) = y(n-1) + x(n) - x(n-N)
      | This requires a careful reset procedure, where the full shift register
      | is zerored out. Otherwise the feedback-based sum stops working.
  RSSI : Inport
  reset : Inport  Port=2
  avglen : Inport  Port=3
  en : Inport  Port=4
  ASR : xbsIndex_r4/Addressable Shift Register  infer_latency=on  depth=2  initVector=[0]  en=on  dbl_ovrd=off  use_behavioral_HDL=off  Optimization=Resource  use_rpm=off  block_type=addrsr
      settings: infoedit="Delay of configurable length.  Any element in the delay line can be addressed and driven onto the output port.<br><br>Hardware notes: This block is implemented using SRL16s. If Virtex-4 or Spartan-3 device is used, multiple SRLC16s are cascaded together."  block_version=VER_STRING_GOES_HERE
  Accumulator : xbsIndex_r4/Accumulator  operation=Add  n_bits=17  overflow=Flag as error  scale=1  rst=on  infoeditControl=reset for floating point data type must be asserted for a minimum of 2 cycles  hasbypass=off  en=on  latency=0  dbl_ovrd=off  msb_inp=100  msb=100  lsb=-100  use_behavioral_HDL=on  implementation=Fabric  block_type=accum
      settings: block_version=VER_STRING_GOES_HERE
  AddSub : xbsIndex_r4/AddSub  mode=Subtraction  use_carryin=off  use_carryout=off  en=off  latency=0  precision=Full  arith_type=Unsigned  n_bits=10  bin_pt=0  quantization=Truncate  overflow=Wrap  dbl_ovrd=off  use_behavioral_HDL=off  hw_selection=Fabric  pipelined=off  use_rpm=on  block_type=addsub
      settings: block_version=VER_STRING_GOES_HERE
  Convert7 : xbsIndex_r4/Convert  gui_display_data_type=Fixed-point  arith_type=Unsigned  n_bits=17  bin_pt=0  float_type=Single  exp_bits=8  fraction_bits=24  quantization=Truncate  overflow=Saturate  en=off  latency=0  dbl_ovrd=off  pipeline=off  block_type=convert
      settings: block_version=10.1.3
  Logical : xbsIndex_r4/Logical  logical_function=OR  inputs=2  en=off  latency=0  precision=Full  arith_type=Unsigned  n_bits=16  bin_pt=0  align_bp=on  dbl_ovrd=off  block_type=logical
  Long Reset Gen : Subsystem
  Register : xbsIndex_r4/Register  init=0  rst=on  en=off  dbl_ovrd=off  block_type=register
      settings: block_version=VER_STRING_GOES_HERE
  avg : Outport
  wires:
  en/1 -> Accumulator/3, ASR/3
  Convert7/1 -> avg/1
  Long Reset Gen/1(reset_out) -> Logical/1
  reset/1 -> Logical/2, Long Reset Gen/2(reset_in)
  Logical/1 -> Accumulator/2, Register/2
  Accumulator/1 -> Convert7/1
  RSSI/1 -> Register/1
  avglen/1 -> Long Reset Gen/1(duration), ASR/2
  Register/1 -> AddSub/1, ASR/1
  AddSub/1 -> Accumulator/1
  ASR/1 -> AddSub/2

== system w3_warplab_trigger_proc/Trigger Sources/Energy/AntC Detector/Busy Detection ==
  Avg RSSI : Inport
  Reset : Inport  Port=2
  en : Inport  Port=3
  Convert1 : xbsIndex_r4/Convert  gui_display_data_type=Fixed-point  arith_type=Unsigned  n_bits=1  bin_pt=0  float_type=Single  exp_bits=8  fraction_bits=24  quantization=Truncate  overflow=Wrap  en=off  latency=0  dbl_ovrd=off  pipeline=off  block_type=convert
      settings: block_version=VER_STRING_GOES_HERE
  Counter1 : xbsIndex_r4/Counter  cnt_type=Free Running  cnt_to=Inf  operation=Up  start_count=0  cnt_by_val=1  arith_type=Unsigned  n_bits=11  bin_pt=0  load_pin=off  rst=on  en=on  explicit_period=off  period=4  dbl_ovrd=off  use_behavioral_HDL=off  implementation=Fabric  use_rpm=off  block_type=counter
  Inverter1 : xbsIndex_r4/Inverter  en=off  latency=0  dbl_ovrd=off  block_type=inv
      settings: xl_area=[0 0 0 0 0 0 0]  block_version=8.2
  Logical : xbsIndex_r4/Logical  logical_function=AND  inputs=2  en=off  latency=0  precision=Full  arith_type=Unsigned  n_bits=16  bin_pt=0  align_bp=on  dbl_ovrd=off  block_type=logical
  Logical1 : xbsIndex_r4/Logical  logical_function=OR  inputs=2  en=off  latency=0  precision=Full  arith_type=Unsigned  n_bits=16  bin_pt=0  align_bp=on  dbl_ovrd=off  block_type=logical
  Relational2 : xbsIndex_r4/Relational  mode=a>b  en=off  latency=0  dbl_ovrd=off  block_type=relational
      settings: block_version=VER_STRING_GOES_HERE
  Relational3 : xbsIndex_r4/Relational  mode=a>b  en=off  latency=0  dbl_ovrd=off  block_type=relational
      settings: block_version=VER_STRING_GOES_HERE
  S-R Latch : Subsystem
  Busy : Outport
  wires:
  [pktDet_energyThresh_busy] -> Relational2/2
  Reset/1 -> Logical1/1
  Logical1/1 -> Counter1/1, S-R Latch/1(R)
  Inverter1/1 -> Logical1/2
  Counter1/1 -> Relational3/1
  [pktDet_duration_busy] -> Relational3/2
  Relational3/1 -> S-R Latch/2(S)
  S-R Latch/1(Q) -> Convert1/1
  Avg RSSI/1 -> Relational2/1
  Convert1/1 -> Busy/1
  Logical/1 -> Counter1/2
  Relational2/1 -> Logical/1, Inverter1/1
  en/1 -> Logical/2

== system w3_warplab_trigger_proc/Trigger Sources/Energy/AntC Detector/Idle Detection ==
  Avg RSSI : Inport
  Reset : Inport  Port=2
  en : Inport  Port=3
  Convert1 : xbsIndex_r4/Convert  gui_display_data_type=Fixed-point  arith_type=Unsigned  n_bits=1  bin_pt=0  float_type=Single  exp_bits=8  fraction_bits=24  quantization=Truncate  overflow=Wrap  en=off  latency=0  dbl_ovrd=off  pipeline=off  block_type=convert
      settings: block_version=VER_STRING_GOES_HERE
  Counter1 : xbsIndex_r4/Counter  cnt_type=Free Running  cnt_to=Inf  operation=Up  start_count=0  cnt_by_val=1  arith_type=Unsigned  n_bits=11  bin_pt=0  load_pin=off  rst=on  en=on  explicit_period=off  period=4  dbl_ovrd=off  use_behavioral_HDL=off  implementation=Fabric  use_rpm=off  block_type=counter
  Inverter1 : xbsIndex_r4/Inverter  en=off  latency=0  dbl_ovrd=off  block_type=inv
      settings: xl_area=[0 0 0 0 0 0 0]  block_version=8.2
  Logical : xbsIndex_r4/Logical  logical_function=AND  inputs=2  en=off  latency=0  precision=Full  arith_type=Unsigned  n_bits=16  bin_pt=0  align_bp=on  dbl_ovrd=off  block_type=logical
  Logical1 : xbsIndex_r4/Logical  logical_function=OR  inputs=2  en=off  latency=0  precision=Full  arith_type=Unsigned  n_bits=16  bin_pt=0  align_bp=on  dbl_ovrd=off  block_type=logical
  Relational2 : xbsIndex_r4/Relational  mode=a<b  en=off  latency=0  dbl_ovrd=off  block_type=relational
      settings: block_version=VER_STRING_GOES_HERE
  Relational3 : xbsIndex_r4/Relational  mode=a>b  en=off  latency=0  dbl_ovrd=off  block_type=relational
      settings: block_version=VER_STRING_GOES_HERE
  S-R Latch : Subsystem
  Idle : Outport
  wires:
  Convert1/1 -> Idle/1
  Avg RSSI/1 -> Relational2/1
  S-R Latch/1(Q) -> Convert1/1
  Relational3/1 -> S-R Latch/2(S)
  [pktDet_duration_idle] -> Relational3/2
  Counter1/1 -> Relational3/1
  Inverter1/1 -> Logical1/2
  Logical1/1 -> Counter1/1, S-R Latch/1(R)
  Reset/1 -> Logical1/1
  Relational2/1 -> Logical/1, Inverter1/1
  [pktDet_energyThresh_idle] -> Relational2/2
  en/1 -> Logical/2
  Logical/1 -> Counter1/2

== system w3_warplab_trigger_proc/Trigger Sources/Energy/AntC Detector/Running Sum ==
  note: This block impelemnts a variable-length running sum.
      | For a sum y(n) of the previous N samples of sequence x(n), it implements
      | y(n) = y(n-1) + x(n) - x(n-N)
      | This requires a careful reset procedure, where the full shift register
      | is zerored out. Otherwise the feedback-based sum stops working.
  RSSI : Inport
  reset : Inport  Port=2
  avglen : Inport  Port=3
  en : Inport  Port=4
  ASR : xbsIndex_r4/Addressable Shift Register  infer_latency=on  depth=2  initVector=[0]  en=on  dbl_ovrd=off  use_behavioral_HDL=off  Optimization=Resource  use_rpm=off  block_type=addrsr
      settings: infoedit="Delay of configurable length.  Any element in the delay line can be addressed and driven onto the output port.<br><br>Hardware notes: This block is implemented using SRL16s. If Virtex-4 or Spartan-3 device is used, multiple SRLC16s are cascaded together."  block_version=VER_STRING_GOES_HERE
  Accumulator : xbsIndex_r4/Accumulator  operation=Add  n_bits=17  overflow=Flag as error  scale=1  rst=on  infoeditControl=reset for floating point data type must be asserted for a minimum of 2 cycles  hasbypass=off  en=on  latency=0  dbl_ovrd=off  msb_inp=100  msb=100  lsb=-100  use_behavioral_HDL=on  implementation=Fabric  block_type=accum
      settings: block_version=VER_STRING_GOES_HERE
  AddSub : xbsIndex_r4/AddSub  mode=Subtraction  use_carryin=off  use_carryout=off  en=off  latency=0  precision=Full  arith_type=Unsigned  n_bits=10  bin_pt=0  quantization=Truncate  overflow=Wrap  dbl_ovrd=off  use_behavioral_HDL=off  hw_selection=Fabric  pipelined=off  use_rpm=on  block_type=addsub
      settings: block_version=VER_STRING_GOES_HERE
  Convert7 : xbsIndex_r4/Convert  gui_display_data_type=Fixed-point  arith_type=Unsigned  n_bits=17  bin_pt=0  float_type=Single  exp_bits=8  fraction_bits=24  quantization=Truncate  overflow=Saturate  en=off  latency=0  dbl_ovrd=off  pipeline=off  block_type=convert
      settings: block_version=10.1.3
  Logical : xbsIndex_r4/Logical  logical_function=OR  inputs=2  en=off  latency=0  precision=Full  arith_type=Unsigned  n_bits=16  bin_pt=0  align_bp=on  dbl_ovrd=off  block_type=logical
  Long Reset Gen : Subsystem
  Register : xbsIndex_r4/Register  init=0  rst=on  en=off  dbl_ovrd=off  block_type=register
      settings: block_version=VER_STRING_GOES_HERE
  avg : Outport
  wires:
  ASR/1 -> AddSub/2
  AddSub/1 -> Accumulator/1
  Register/1 -> ASR/1, AddSub/1
  avglen/1 -> ASR/2, Long Reset Gen/1(duration)
  RSSI/1 -> Register/1
  Accumulator/1 -> Convert7/1
  Logical/1 -> Register/2, Accumulator/2
  reset/1 -> Long Reset Gen/2(reset_in), Logical/2
  Long Reset Gen/1(reset_out) -> Logical/1
  Convert7/1 -> avg/1
  en/1 -> ASR/3, Accumulator/3

== system w3_warplab_trigger_proc/Trigger Sources/Energy/AntD Detector/Busy Detection ==
  Avg RSSI : Inport
  Reset : Inport  Port=2
  en : Inport  Port=3
  Convert1 : xbsIndex_r4/Convert  gui_display_data_type=Fixed-point  arith_type=Unsigned  n_bits=1  bin_pt=0  float_type=Single  exp_bits=8  fraction_bits=24  quantization=Truncate  overflow=Wrap  en=off  latency=0  dbl_ovrd=off  pipeline=off  block_type=convert
      settings: block_version=VER_STRING_GOES_HERE
  Counter1 : xbsIndex_r4/Counter  cnt_type=Free Running  cnt_to=Inf  operation=Up  start_count=0  cnt_by_val=1  arith_type=Unsigned  n_bits=11  bin_pt=0  load_pin=off  rst=on  en=on  explicit_period=off  period=4  dbl_ovrd=off  use_behavioral_HDL=off  implementation=Fabric  use_rpm=off  block_type=counter
  Inverter1 : xbsIndex_r4/Inverter  en=off  latency=0  dbl_ovrd=off  block_type=inv
      settings: xl_area=[0 0 0 0 0 0 0]  block_version=8.2
  Logical : xbsIndex_r4/Logical  logical_function=AND  inputs=2  en=off  latency=0  precision=Full  arith_type=Unsigned  n_bits=16  bin_pt=0  align_bp=on  dbl_ovrd=off  block_type=logical
  Logical1 : xbsIndex_r4/Logical  logical_function=OR  inputs=2  en=off  latency=0  precision=Full  arith_type=Unsigned  n_bits=16  bin_pt=0  align_bp=on  dbl_ovrd=off  block_type=logical
  Relational2 : xbsIndex_r4/Relational  mode=a>b  en=off  latency=0  dbl_ovrd=off  block_type=relational
      settings: block_version=VER_STRING_GOES_HERE
  Relational3 : xbsIndex_r4/Relational  mode=a>b  en=off  latency=0  dbl_ovrd=off  block_type=relational
      settings: block_version=VER_STRING_GOES_HERE
  S-R Latch : Subsystem
  Busy : Outport
  wires:
  [pktDet_energyThresh_busy] -> Relational2/2
  Reset/1 -> Logical1/1
  Logical1/1 -> Counter1/1, S-R Latch/1(R)
  Inverter1/1 -> Logical1/2
  Counter1/1 -> Relational3/1
  [pktDet_duration_busy] -> Relational3/2
  Relational3/1 -> S-R Latch/2(S)
  S-R Latch/1(Q) -> Convert1/1
  Avg RSSI/1 -> Relational2/1
  Convert1/1 -> Busy/1
  Logical/1 -> Counter1/2
  Relational2/1 -> Logical/1, Inverter1/1
  en/1 -> Logical/2
